simulink model "DiffEq2_Model"  (R2025b)
settings: Solver=FixedStepDiscrete  StartTime=0.0  StopTime=20  FixedStep=1  RelTol=1e-3
settings Model: Creator=Rashid  LastModifiedBy=Rashid

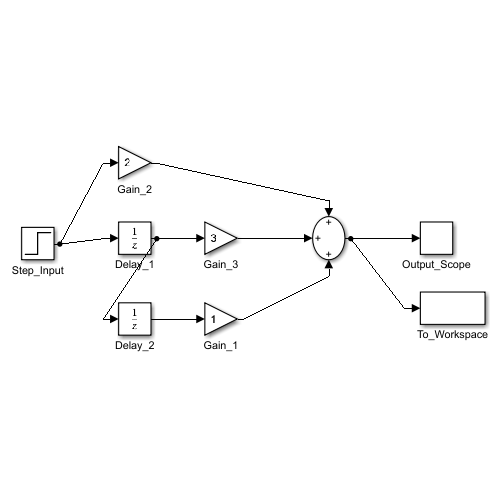
[thumbnail: Simulink's stored preview of the top-level diagram]
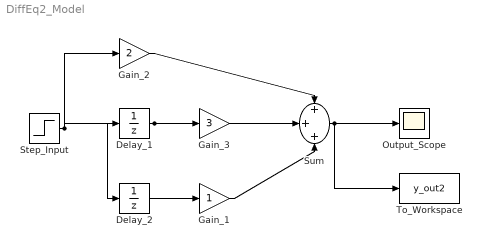
== system DiffEq2_Model ==
  Delay_1 : UnitDelay  HasFrameUpgradeWarning=on
  Delay_2 : UnitDelay  HasFrameUpgradeWarning=on
  Gain_1 : Gain
  Gain_2 : Gain  Gain=2
  Gain_3 : Gain  Gain=3
  Output_Scope : Scope
  Step_Input : Step  Time=0  SampleTime=0
  Sum : Sum  Inputs=+++
  To_Workspace : ToWorkspace  VariableName=y_out2  SampleTime=-1
  wires:
  Step_Input/1 -> Gain_2/1, Delay_1/1
  Delay_1/1 -> Gain_3/1, Delay_2/1
  Delay_2/1 -> Gain_1/1
  Gain_2/1 -> Sum/1
  Gain_3/1 -> Sum/2
  Gain_1/1 -> Sum/3
  Sum/1 -> Output_Scope/1, To_Workspace/1
